simulink model "decoupleController"  (R2021a)
settings: Solver=VariableStepAuto  StartTime=0.0  StopTime=10.0  RelTol=1e-3
values from neighbouring files (symbols this model uses):
  A_A = f_AA3    [SupportFile.m]
  A_E = F_AE3    [SupportFile.m]
  A_R = f_AR2    [SupportFile.m]
  A_T = f_At1    [SupportFile.m]
  B_A = f_BA1    [SupportFile.m]
  B_E = f_BE1    [SupportFile.m]
  B_R = f_BR1    [SupportFile.m]
  B_T = f_Bt1    [SupportFile.m]
  C_A = eye(3)    [SupportFile.m]
  C_E = eye(3)    [SupportFile.m]
  C_R = eye(2)    [SupportFile.m]
  C_T = eye(2)    [SupportFile.m]
  D_A = zeros(3,1)    [SupportFile.m]
  D_E = zeros(3,1)    [SupportFile.m]
  D_R = zeros(2,1)    [SupportFile.m]
  D_T = zeros(2,1)    [SupportFile.m]
  K_A = place(A_A, B_A, [-5 -2 -1])    [SupportFile.m]
  K_E = place(A_E, B_E, [-5 -2 -1])    [SupportFile.m]
  K_R = place(A_R, B_R, [-5 -2])    [SupportFile.m]
  K_T = place(A_T, B_T, [-5 -2])    [SupportFile.m]
settings Model: Creator=jiasen.z  LastModifiedBy=jiasen.z

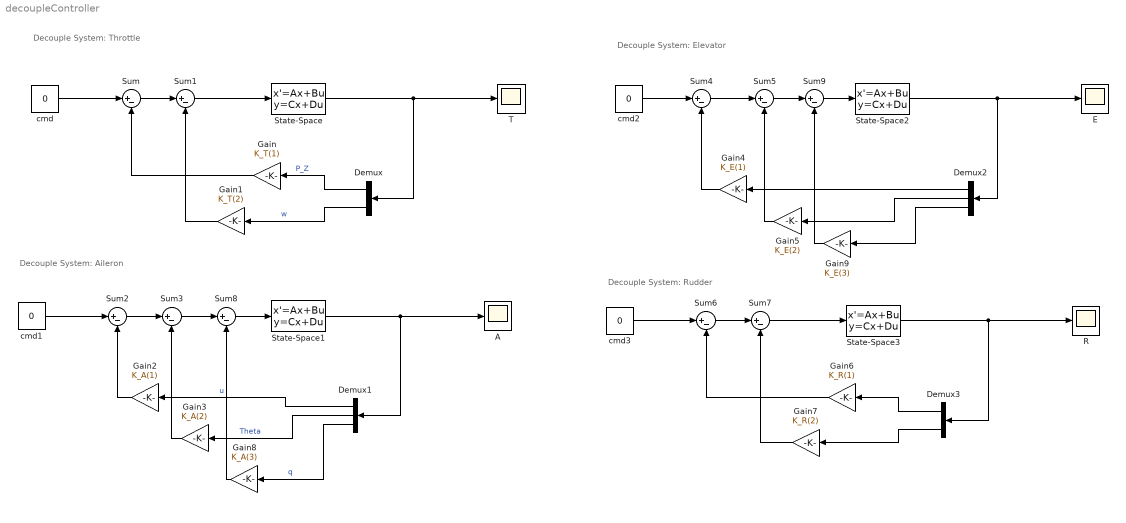
== system decoupleController ==
  note: Decouple System: Throttle
  note: Decouple System: Aileron
  note: Decouple System: Elevator
  note: Decouple System: Rudder
  A : Scope
  Demux : Demux  Outputs=2
  Demux1 : Demux  Outputs=3
  Demux2 : Demux  Outputs=3
  Demux3 : Demux  Outputs=2
  E : Scope
  Gain : Gain  Gain=K_T(1)
  Gain1 : Gain  Gain=K_T(2)
  Gain2 : Gain  Gain=K_A(1)
  Gain3 : Gain  Gain=K_A(2)
  Gain4 : Gain  Gain=K_E(1)
  Gain5 : Gain  Gain=K_E(2)
  Gain6 : Gain  Gain=K_R(1)
  Gain7 : Gain  Gain=K_R(2)
  Gain8 : Gain  Gain=K_A(3)
  Gain9 : Gain  Gain=K_E(3)
  R : Scope
  State-Space : StateSpace  A=A_T  B=B_T  C=C_T  D=D_T  InitialCondition=[1,1]
  State-Space1 : StateSpace  A=A_A  B=B_A  C=C_A  D=D_A  InitialCondition=[1,1,1]
  State-Space2 : StateSpace  A=A_E  B=B_E  C=C_E  D=D_E  InitialCondition=[1,1,1]
  State-Space3 : StateSpace  A=A_R  B=B_R  C=C_R  D=D_R  InitialCondition=[1,1]
  Sum{,1..9} (10 alike) : Sum  Inputs=|+-
  T : Scope
  cmd{,1..3} (4 alike) : Constant  Value=0
  wires:
  Sum1/1 -> State-Space/1
  Sum/1 -> Sum1/1
  cmd/1 -> Sum/1
  State-Space/1 -> Demux/1, T/1
  Demux/1 -> Gain/1  "P_Z"
  Gain/1 -> Sum/2
  Demux/2 -> Gain1/1  "w"
  Gain1/1 -> Sum1/2
  Sum2/1 -> Sum3/1
  Demux1/2 -> Gain3/1  "Theta"
  Gain2/1 -> Sum2/2
  cmd1/1 -> Sum2/1
  State-Space1/1 -> Demux1/1, A/1
  Gain3/1 -> Sum3/2
  Demux1/1 -> Gain2/1  "u"
  Sum4/1 -> Sum5/1
  Demux2/2 -> Gain5/1
  Gain4/1 -> Sum4/2
  cmd2/1 -> Sum4/1
  State-Space2/1 -> Demux2/1, E/1
  Gain5/1 -> Sum5/2
  Demux2/1 -> Gain4/1
  Sum6/1 -> Sum7/1
  Demux3/2 -> Gain7/1
  Gain6/1 -> Sum6/2
  cmd3/1 -> Sum6/1
  State-Space3/1 -> Demux3/1, R/1
  Gain7/1 -> Sum7/2
  Demux3/1 -> Gain6/1
  Sum7/1 -> State-Space3/1
  Sum8/1 -> State-Space1/1
  Sum3/1 -> Sum8/1
  Gain8/1 -> Sum8/2
  Demux1/3 -> Gain8/1  "q"
  Sum5/1 -> Sum9/1
  Sum9/1 -> State-Space2/1
  Gain9/1 -> Sum9/2
  Demux2/3 -> Gain9/1
